simulink model "Strategia_pilotaggio_XY"  (R2020b)
settings: Solver=VariableStepAuto  StartTime=0.0  StopTime=tsim  RelTol=1e-3
values from neighbouring files (symbols this model uses):
  Acc_asse_x = []    [main_Strategia_di_pilotaggio.m]
  Acc_asse_y = []    [main_Strategia_di_pilotaggio.m]
  mx = config_dc_x(parx)    [Main_traiettoria.m]    (also in Main_traiettoria_ordinato.m; main_Strategia_di_pilotaggio.m)
  my = config_dc_y(pary)    [Main_traiettoria.m]    (also in Main_traiettoria_ordinato.m; main_Strategia_di_pilotaggio.m)
  time = 0:tf/np:tf    [Main_traiettoria.m]    (also in Main_traiettoria_ordinato.m = 0:passo:tsim)
  Vel_asse_x = []    [main_Strategia_di_pilotaggio.m]
  Vel_asse_y = []    [main_Strategia_di_pilotaggio.m]
  x = zeros(length(time),1)    [Main_traiettoria.m]    (also in Main_traiettoria_ordinato.m; main_Strategia_di_pilotaggio.m = [])
  y = zeros(length(time),1)    [Main_traiettoria.m]    (also in Main_traiettoria_ordinato.m; main_Strategia_di_pilotaggio.m = [])
undefined symbols (not defined in the file or in its folder): accelerazioni, accelerazioniy, ci_x, ci_y, Evaluate_Trajectory, interpolazione_tempi, parx, pary
libraries: cstblocks x16, simulink x3
settings Model: Creator=stefa  LastModifiedBy=user
settings DebuggingCC: SFMachineParentedDataDiag=error

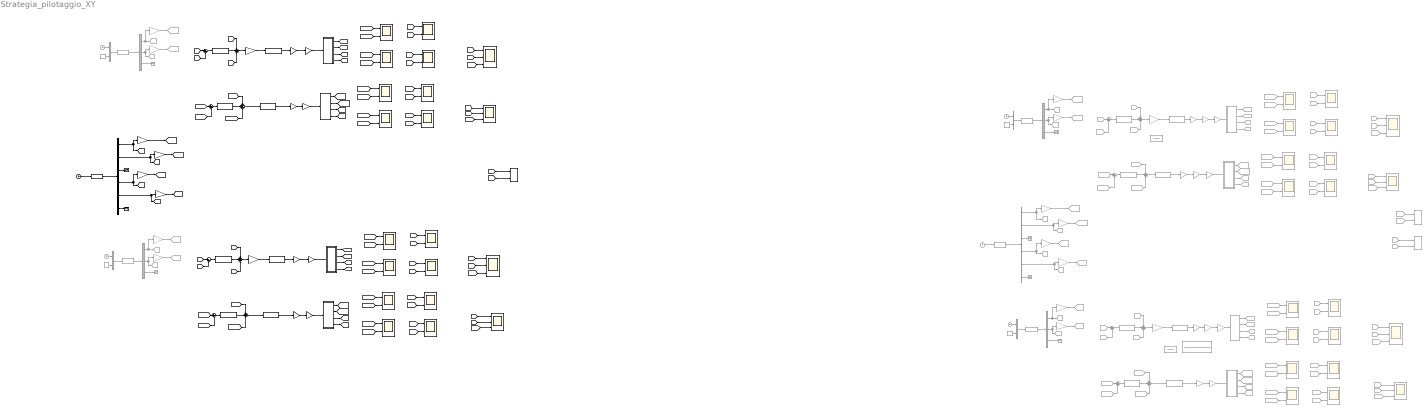
== system Strategia_pilotaggio_XY ==
  note: Vel carrello confronto
  note: Retroazione Motore
  note: Retroazione Motore
  note: Grafici
  note: Grafici
  note: Retroazione carrello
  note: ASSE "X"
  note: Pos carrello confronto
  note: Retroazione carrello
  note: Pos carrello confronto
  note: ASSE "Y"
  note: Vel carrello confronto
  note: ASSE "XY"
  note: Retroazione Motore
  note: Grafici
  note: Vel carrello confronto
  note: Grafici
  note: ASSE "Y"
  note: Pos carrello confronto
  note: Retroazione Motore
  note: Retroazione carrello
  note: Pos carrello confronto
  note: Retroazione carrello
  note: ASSE "XY"
  note: Vel carrello confronto
  note: ASSE "X"
   {1..2,5..8} (6 alike) : Terminator  Commented=on
  " 3" : Terminator
  " 4" : Terminator
  Constant{1..4} (4 alike) : Constant  Commented=on  Value=0.6
  Demux{1..2,4..5} (4 alike) : Demux  Commented=on  Outputs=3
  Demux3 : Demux  Outputs=6
  Demux6 : Demux  Commented=on  Outputs=6
  Discrete Filter1 : DiscreteFilter  Commented=on  Denominator=[1 0.7]
  Discrete Filter2 : DiscreteFilter  Commented=on  Denominator=[1 0.3]
  Discrete Filter3 : DiscreteFilter  Commented=on  Denominator=[(2*pi*150)^2 (2*pi*150/0.8) 1]
  From{100,107,110,119} (4 alike) : From  Commented=on  GotoTag=y
  From101 : From  Commented=on  GotoTag=theta1_ref
  From102 : From  Commented=on  GotoTag=theta1_rifmot
  From103 : From  Commented=on  GotoTag=theta1p_ref
  From104 : From  Commented=on  GotoTag=theta1p_rifmot
  From{87,98,105,112} (4 alike) : From  Commented=on  GotoTag=y_ref
  From{63,73,81,106} (4 alike) : From  Commented=on  GotoTag=x_ref
  From{99,108,114..115} (4 alike) : From  Commented=on  GotoTag=yp_ref
  From109 : From  Commented=on  GotoTag=yp
  From111 : From  Commented=on  GotoTag=yp_rifmot
  From113 : From  Commented=on  GotoTag=y_rifmot
  From116 : From  Commented=on  GotoTag=x_rifmot
  From117 : From  Commented=on  GotoTag=yp
  From{76,82,96,118} (4 alike) : From  Commented=on  GotoTag=x
  From{75,83,120..121} (4 alike) : From  Commented=on  GotoTag=xp_ref
  From122 : From  Commented=on  GotoTag=xp
  From123 : From  Commented=on  GotoTag=xp
  From124 : From  Commented=on  GotoTag=theta1p_rifmotx
  From125 : From  Commented=on  GotoTag=yp
  From126 : From  Commented=on  GotoTag=theta1p_rifmot
  From64 : From  Commented=on  GotoTag=xp_rifmot
  From65 : From  Commented=on  GotoTag=theta1_refx
  From66 : From  Commented=on  GotoTag=theta1p_refx
  From67 : From  Commented=on  GotoTag=theta1_rifmotx
  From68 : From  Commented=on  GotoTag=theta1_refx
  From69 : From  Commented=on  GotoTag=theta1x
  From70 : From  Commented=on  GotoTag=theta1p_refx
  From71 : From  Commented=on  GotoTag=theta1px
  From72 : From  Commented=on  GotoTag=x_rifmot
  From74 : From  Commented=on  GotoTag=x_rifmot
  From77 : From  Commented=on  GotoTag=theta1_refx
  From78 : From  Commented=on  GotoTag=theta1_rifmotx
  From79 : From  Commented=on  GotoTag=theta1p_refx
  From80 : From  Commented=on  GotoTag=theta1p_rifmotx
  From84 : From  Commented=on  GotoTag=xp
  From85 : From  Commented=on  GotoTag=y_rifmot
  From86 : From  Commented=on  GotoTag=xp_rifmot
  From88 : From  Commented=on  GotoTag=yp_rifmot
  From89 : From  Commented=on  GotoTag=theta1_ref
  From90 : From  Commented=on  GotoTag=theta1p_ref
  From91 : From  Commented=on  GotoTag=theta1_rifmot
  From92 : From  Commented=on  GotoTag=theta1_ref
  From93 : From  Commented=on  GotoTag=theta1
  From94 : From  Commented=on  GotoTag=theta1p_ref
  From95 : From  Commented=on  GotoTag=theta1p
  From97 : From  Commented=on  GotoTag=y_rifmot
  G-agg : Gain  Commented=on  Gain=0.09
  G_AGG : Gain  Commented=on  Gain=0.5
  G_AGG1 : Gain  Commented=on  Gain=0.19
  Gain{1,4,11,13,15,18..19} (7 alike) : Gain  Commented=on  Gain=1/parx.tau
  Gain10 : Gain  Gain=1/pary.tau
  Gain{3,6,12,14,16..17,20} (7 alike) : Gain  Commented=on  Gain=1/pary.tau
  Gain2 : Gain  Gain=1/parx.tau
  Gain5 : Gain  Gain=1/pary.tau
  Gain7 : Gain  Gain=1/parx.tau
  Gain8 : Gain  Gain=1/parx.tau
  Gain9 : Gain  Gain=1/pary.tau
  Goto11 : Goto  Commented=on  GotoTag=xp_ref
  Goto14 : Goto  Commented=on  GotoTag=yp_ref
  Goto18 : Goto  Commented=on  GotoTag=theta1_ref
  Goto2 : Goto  Commented=on  GotoTag=theta1_refx
  Goto20 : Goto  Commented=on  GotoTag=theta1p_ref
  Goto23 : Goto  Commented=on  GotoTag=y_ref
  Goto33 : Goto  Commented=on  GotoTag=xp_rifmot
  Goto34 : Goto  Commented=on  GotoTag=xp
  Goto35 : Goto  Commented=on  GotoTag=xp_ref
  Goto36 : Goto  Commented=on  GotoTag=yp
  Goto37 : Goto  Commented=on  GotoTag=theta1p_rifmotx
  Goto38 : Goto  Commented=on  GotoTag=yp_ref
  Goto39 : Goto  Commented=on  GotoTag=x
  Goto4 : Goto  Commented=on  GotoTag=theta1p_refx
  Goto40 : Goto  Commented=on  GotoTag=theta1p_rifmot
  Goto41 : Goto  Commented=on  GotoTag=y
  Goto42 : Goto  Commented=on  GotoTag=theta1_ref
  Goto43 : Goto  Commented=on  GotoTag=y_rifmot
  Goto44 : Goto  Commented=on  GotoTag=theta1_refx
  Goto45 : Goto  Commented=on  GotoTag=theta1p_ref
  Goto46 : Goto  Commented=on  GotoTag=theta1p
  Goto47 : Goto  Commented=on  GotoTag=theta1
  Goto48 : Goto  Commented=on  GotoTag=y_ref
  Goto49 : Goto  Commented=on  GotoTag=theta1_rifmot
  Goto50 : Goto  Commented=on  GotoTag=xp_ref
  Goto51 : Goto  Commented=on  GotoTag=theta1_refx
  Goto52 : Goto  Commented=on  GotoTag=theta1p_refx
  Goto53 : Goto  Commented=on  GotoTag=x_ref
  Goto54 : Goto  Commented=on  GotoTag=yp_ref
  Goto55 : Goto  Commented=on  GotoTag=x_rifmot
  Goto56 : Goto  Commented=on  GotoTag=theta1_ref
  Goto57 : Goto  Commented=on  GotoTag=theta1p_ref
  Goto58 : Goto  Commented=on  GotoTag=y_ref
  Goto59 : Goto  Commented=on  GotoTag=theta1p_refx
  Goto60 : Goto  Commented=on  GotoTag=theta1px
  Goto61 : Goto  Commented=on  GotoTag=theta1x
  Goto62 : Goto  Commented=on  GotoTag=yp_rifmot
  Goto63 : Goto  Commented=on  GotoTag=x_ref
  Goto64 : Goto  Commented=on  GotoTag=theta1_rifmotx
  Goto8 : Goto  Commented=on  GotoTag=x_ref
  Km : Gain  Gain=mx.K
  Km1 : Gain  Gain=my.K
  Km2 : Gain  Commented=on  Gain=mx.K
  Km3 : Gain  Commented=on  Gain=my.K
  Kr : Gain  Gain=mx.Kr
  Kr1 : Gain  Gain=mx.Kr
  Kr2 : Gain  Gain=my.Kr
  Kr3 : Gain  Gain=my.Kr
  Kr4 : Gain  Commented=on  Gain=mx.Kr
  Kr5 : Gain  Commented=on  Gain=mx.Kr
  Kr6 : Gain  Commented=on  Gain=my.Kr
  Kr7 : Gain  Commented=on  Gain=my.Kr
  Mux{1..4} (4 alike) : Mux  Commented=on  Inputs=2
  Pos. Motore con retr. Mot : Scope  NumInputPorts=2
  Pos. Motore con retr. Mot1 : Scope  NumInputPorts=2
  Pos. Motore con retr. Mot2 : Scope  Commented=on  NumInputPorts=2
  Pos. Motore con retr. Mot3 : Scope  Commented=on  NumInputPorts=2
  Pos. Motore con retr. carrello : Scope  NumInputPorts=2
  Pos. Motore con retr. carrello1 : Scope  NumInputPorts=2
  Pos. Motore con retr. carrello2 : Scope  Commented=on  NumInputPorts=2
  Pos. Motore con retr. carrello3 : Scope  Commented=on  NumInputPorts=2
  Pos. carrello con retr. Mot : Scope  NumInputPorts=2
  Pos. carrello con retr. Mot1 : Scope  NumInputPorts=2
  Pos. carrello con retr. Mot2 : Scope  Commented=on  NumInputPorts=2
  Pos. carrello con retr. Mot3 : Scope  Commented=on  NumInputPorts=2
  Pos. carrello con retr. carrello : Scope  NumInputPorts=2
  Pos. carrello con retr. carrello1 : Scope  NumInputPorts=2
  Pos. carrello con retr. carrello2 : Scope  Commented=on  NumInputPorts=2
  Pos. carrello con retr. carrello3 : Scope  Commented=on  NumInputPorts=2
  Pos. carrello confronto : Scope  NumInputPorts=3
  Pos. carrello confronto1 : Scope  NumInputPorts=3
  Pos. carrello confronto2 : Scope  Commented=on  NumInputPorts=3
  Pos. carrello confronto3 : Scope  Commented=on  NumInputPorts=3
  REGOLATORE POSIZIONE1 : cstblocks/LTI System  sys=apx.H_P  IC=[]
  REGOLATORE POSIZIONE2 : cstblocks/LTI System  sys=apx.H_P  IC=[]
  REGOLATORE POSIZIONE3 : cstblocks/LTI System  sys=apy.H_P  IC=[]
  REGOLATORE POSIZIONE4 : cstblocks/LTI System  sys=apy.H_P  IC=[]
  REGOLATORE POSIZIONE5 : cstblocks/LTI System  Commented=on  sys=apx.H_P  IC=[]
  REGOLATORE POSIZIONE6 : cstblocks/LTI System  Commented=on  sys=apx.H_P  IC=[]
  REGOLATORE POSIZIONE7 : cstblocks/LTI System  Commented=on  sys=apy.H_P  IC=[]
  REGOLATORE POSIZIONE8 : cstblocks/LTI System  Commented=on  sys=apy.H_P  IC=[]
  REGOLATORE VELOCITA1 : cstblocks/LTI System  sys=avx.PI_V  IC=[]
  REGOLATORE VELOCITA2 : cstblocks/LTI System  sys=avx.PI_V  IC=[]
  REGOLATORE VELOCITA3 : cstblocks/LTI System  sys=avy.PI_V  IC=[]
  REGOLATORE VELOCITA4 : cstblocks/LTI System  sys=avy.PI_V  IC=[]
  REGOLATORE VELOCITA5 : cstblocks/LTI System  Commented=on  sys=avx.PI_V  IC=[]
  REGOLATORE VELOCITA6 : cstblocks/LTI System  Commented=on  sys=avx.PI_V  IC=[]
  REGOLATORE VELOCITA7 : cstblocks/LTI System  Commented=on  sys=avy.PI_V  IC=[]
  REGOLATORE VELOCITA8 : cstblocks/LTI System  Commented=on  sys=avy.PI_V  IC=[]
  Sum{1..2,5..6} (4 alike) : Sum  Inputs=|+-
  Sum{9..10,13..14} (4 alike) : Sum  Commented=on  Inputs=|+-
  Sum{11..12,15..16} (4 alike) : Sum  Commented=on  Inputs=++-
  Sum{3..4,7..8} (4 alike) : Sum  Inputs=++-
  Vel. Motore con retr. Mot : Scope  NumInputPorts=2
  Vel. Motore con retr. Mot1 : Scope  NumInputPorts=2
  Vel. Motore con retr. Mot2 : Scope  Commented=on  NumInputPorts=2
  Vel. Motore con retr. Mot3 : Scope  Commented=on  NumInputPorts=2
  Vel. Motore con retr. carrello : Scope  NumInputPorts=2
  Vel. Motore con retr. carrello1 : Scope  NumInputPorts=2
  Vel. Motore con retr. carrello2 : Scope  Commented=on  NumInputPorts=2
  Vel. Motore con retr. carrello3 : Scope  Commented=on  NumInputPorts=2
  Vel. carrello con retr. Mot : Scope  NumInputPorts=2
  Vel. carrello con retr. Mot1 : Scope  NumInputPorts=2
  Vel. carrello con retr. Mot2 : Scope  Commented=on  NumInputPorts=2
  Vel. carrello con retr. Mot3 : Scope  Commented=on  NumInputPorts=2
  Vel. carrello con retr. carrello : Scope  NumInputPorts=2
  Vel. carrello con retr. carrello1 : Scope  NumInputPorts=2
  Vel. carrello con retr. carrello2 : Scope  Commented=on  NumInputPorts=2
  Vel. carrello con retr. carrello3 : Scope  Commented=on  NumInputPorts=2
  Vel. carrello confronto : Scope  NumInputPorts=3
  Vel. carrello confronto1 : Scope  NumInputPorts=3
  Vel. carrello confronto2 : Scope  Commented=on  NumInputPorts=3
  Vel. carrello confronto3 : Scope  Commented=on  NumInputPorts=3
  XY Graph : simulink/Sinks/XY Graph  xmin=-1  xmax=1  ymin=-1  ymax=1  st=-1
  XY Graph1 : simulink/Sinks/XY Graph  Commented=on  xmin=-0.5  xmax=0.3  ymin=-0.5  ymax=0.3  st=-1
  XY Graph2 : simulink/Sinks/XY Graph  Commented=on  xmin=-0.5  xmax=0.3  ymin=-0.5  ymax=0.3  st=-1
  blocco 4 gdl1 : Subsystem
  blocco 4 gdl2 : Subsystem
  blocco 4 gdl3 : Subsystem
  blocco 4 gdl4 : Subsystem
  blocco 4 gdl5 : Subsystem  Commented=on
  blocco 4 gdl6 : Subsystem  Commented=on
  blocco 4 gdl7 : Subsystem  Commented=on
  blocco 4 gdl8 : Subsystem  Commented=on
  chopper1 : Gain  Gain=my.K
  chopper2 : Gain  Gain=mx.K
  chopper3 : Gain  Commented=on  Gain=my.K
  chopper4 : Gain  Commented=on  Gain=mx.K
  generatore profilo moto{1..2,4..5} (4 alike) : MATLABFcn  Commented=on  MATLABFcn=Evaluate_Trajectory( u(1) , u(2))  OutputDimensions=3
  generatore profilo moto3 : MATLABFcn  MATLABFcn=interpolazione_tempi(x,Vel_asse_x,Acc_asse_x,y,Vel_asse_y,Acc_asse_y,u,time)  OutputDimensions=6
  generatore profilo moto6 : MATLABFcn  Commented=on  MATLABFcn=interpolazione_tempi(x,Vel_asse_x,Acc_asse_x,y,Vel_asse_y,Acc_asse_y,u,time)  OutputDimensions=6
  tempo{1..2,4..6} (5 alike) : Clock  Commented=on
      tempo6 settings: Decimation=tsim
  tempo3 : Clock
      settings: Decimation=tsim
  wires:
  [y] -> XY Graph/2  "y retr. carrello"
  [theta1p] -> Vel. Motore con retr. carrello1/2  "theta1p"
  Mux2/1 -> generatore profilo moto1/1
  [theta1p_ref] -> Vel. Motore con retr. carrello1/1  "thehta1p_ref"
  Mux1/1 -> generatore profilo moto2/1
  [theta1_rifmot] -> Sum5/2
  blocco 4 gdl4/2(Out1) -> [theta1p_rifmot]
  [xp] -> Vel. carrello confronto/2  "xp_retcarr"
  Demux3/2 -> Gain7/1, [xp_ref]  "XP"
  [yp_rifmot] -> Vel. carrello con retr. Mot1/2  "yp"
  [theta1p_refx] -> Vel. Motore con retr. Mot/1  "theta1p_ref"
  tempo1/1 -> Mux2/1
  blocco 4 gdl3/1(Out2) -> [theta1]
  Demux3/5 -> Gain9/1, [yp_ref]  "YP"
  [yp_ref] -> Sum7/1
  [x] -> XY Graph/1  "x_retcarr"
  Gain10/1 -> [theta1_ref]  "motore"
  [theta1p_rifmot] -> Vel. Motore con retr. Mot1/2  "theta1p"
  [theta1p_ref] -> Sum8/1
  [y_ref] -> Pos. carrello con retr. carrello1/1  "y_ref"
  Demux3/3 -> " 3"/1  "XPP"
  Demux1/2 -> Gain3/1, Goto14/1  "YP"
  Gain9/1 -> [theta1p_ref]  "motore"
  tempo3/1 -> generatore profilo moto3/1
  Demux3/4 -> Gain10/1, [y_ref]  "Y"
  Demux3/6 -> " 4"/1  "YPP"
  Km1/1 -> blocco 4 gdl3/1(In1)  "Cm"
  [x_ref] -> Pos. carrello con retr. carrello/1  "x_ref"
  [y_rifmot] -> Pos. carrello con retr. Mot1/2  "y"
  blocco 4 gdl4/3(Out3) -> [y_rifmot]
  blocco 4 gdl2/2(Out4) -> [theta1p_rifmotx]
  blocco 4 gdl3/2(Out1) -> [theta1p]
  [theta1_rifmot] -> Pos. Motore con retr. Mot1/2  "theta1"
  [y_ref] -> Pos. carrello con retr. Mot1/1  "y_ref"
  Kr2/1 -> Km1/1  "I"
  [y_ref] -> Pos. carrello confronto1/1  "y ldm"
  Gain8/1 -> [theta1_refx]  "motore"
  Demux3/1 -> Gain8/1, [x_ref]  "X"
  Gain7/1 -> [theta1p_refx]  "motore"
  REGOLATORE POSIZIONE4/1 -> Sum8/2
  [y] -> Sum6/2
  [theta1_rifmotx] -> Pos. Motore con retr. Mot/2  "theta1"
  [theta1_ref] -> Pos. Motore con retr. carrello1/1  "theta1_ref"
  [theta1_rifmotx] -> Sum1/2
  blocco 4 gdl3/3(Out3) -> [y]
  [y] -> Pos. carrello con retr. carrello1/2  "y"
  Constant1/1 -> Mux1/2
  Sum3/1 -> Gain2/1
  [yp] -> Sum7/3
  [y_ref] -> Sum6/1
  blocco 4 gdl4/1(Out2) -> [theta1_rifmot]
  Sum5/1 -> REGOLATORE POSIZIONE4/1
  [x] -> Pos. carrello confronto/2  "x_retcarr"
  Gain3/1 -> Goto20/1  "motore"
  blocco 4 gdl1/4(Out8) -> [xp]
  [theta1p_rifmot] -> Sum8/3
  [yp_ref] -> Vel. carrello con retr. Mot1/1  "yp_ref"
  Constant2/1 -> Mux2/2
  REGOLATORE POSIZIONE3/1 -> Sum7/2
  Gain6/1 -> Goto18/1  "motore"
  [yp_ref] -> Vel. carrello con retr. carrello1/1  "yp_ref"
  [xp_ref] -> Vel. carrello con retr. carrello/1  "xp_ref"
  Sum6/1 -> REGOLATORE POSIZIONE3/1
  [theta1_refx] -> Sum1/1
  [yp] -> Vel. carrello con retr. carrello1/2  "yp"
  [xp_ref] -> Vel. carrello con retr. Mot/1  "xp_ref"
  REGOLATORE VELOCITA4/1 -> Kr2/1  "Va"
  REGOLATORE VELOCITA3/1 -> Kr3/1  "Va"
  Sum8/1 -> REGOLATORE VELOCITA3/1
  [yp_rifmot] -> Vel. carrello confronto1/3  "yp retr. motore"
  generatore profilo moto1/1 -> Demux1/1  "carrello"
  [xp_rifmot] -> Vel. carrello confronto/3  "xp_retmot"
  blocco 4 gdl3/4(Out4) -> [yp]
  [theta1x] -> Pos. Motore con retr. carrello/2  "tetha1"
  [y] -> Pos. carrello confronto1/2  "y retr. carrello"
  [xp] -> Sum3/3
  [theta1p_ref] -> Vel. Motore con retr. Mot1/1  "thehta1p_ref"
  Demux1/3 -> " 2"/1  "YPP"
  blocco 4 gdl1/1(Out3) -> [theta1x]
  Gain5/1 -> REGOLATORE VELOCITA4/1  "theta1_rif"
  chopper2/1 -> blocco 4 gdl2/1(In1)  "Cm"
  [theta1] -> Pos. Motore con retr. carrello1/2  "theta1"
  blocco 4 gdl1/3(Out7) -> [x]
  Gain1/1 -> Goto4/1  "motore"
  [x_ref] -> Pos. carrello confronto/1  "x_ref"
  [xp_ref] -> Vel. carrello confronto/1  "xp_ref"
  Gain4/1 -> Goto2/1  "motore"
  Sum1/1 -> REGOLATORE POSIZIONE2/1
  [theta1p_rifmotx] -> Sum4/3
  [x_ref] -> Pos. carrello con retr. Mot/1  "x"
  REGOLATORE POSIZIONE2/1 -> Sum4/2
  [x_rifmot] -> Pos. carrello con retr. Mot/2  "x_rif"
  [theta1_refx] -> Pos. Motore con retr. carrello/1  "theta1_ref"
  REGOLATORE VELOCITA1/1 -> Kr1/1  "Va"
  [theta1p_rifmotx] -> Vel. Motore con retr. Mot/2  "theta1p"
  [theta1p_refx] -> Vel. Motore con retr. carrello/1  "theta1p_ref"
  Km/1 -> blocco 4 gdl1/1(In1)  "Cm"
  [x] -> Sum2/2
  [theta1_refx] -> Pos. Motore con retr. Mot/1  "theta1_ref"
  Demux2/2 -> Gain1/1, Goto11/1  "XP"
  Sum7/1 -> Gain5/1
  blocco 4 gdl1/2(Out4) -> [theta1px]
  [xp] -> Vel. carrello con retr. carrello/2  "xp"
  [x_ref] -> Sum2/1
  Demux2/1 -> Goto8/1, Gain4/1  "X"
  [theta1_ref] -> Pos. Motore con retr. Mot1/1  "theta1_ref"
  generatore profilo moto2/1 -> Demux2/1  "carrello"
  [theta1px] -> Vel. Motore con retr. carrello/2  "thehta1p"
  tempo2/1 -> Mux1/1
  Gain2/1 -> REGOLATORE VELOCITA2/1  "theta1_rifx"
  generatore profilo moto3/1 -> Demux3/1  "carrello"
  [yp] -> Vel. carrello confronto1/2  "yp retr. carrello"
  Kr1/1 -> chopper2/1  "I"
  Demux2/3 -> " 1"/1  "XPP"
  [xp_ref] -> Sum3/1
  Kr/1 -> Km/1  "I"
  Sum4/1 -> REGOLATORE VELOCITA1/1
  REGOLATORE POSIZIONE1/1 -> Sum3/2
  REGOLATORE VELOCITA2/1 -> Kr/1  "Va"
  [theta1p_refx] -> Sum4/1
  blocco 4 gdl2/3(Out7) -> [x_rifmot]
  blocco 4 gdl2/4(Out1) -> [xp_rifmot]
  Kr3/1 -> chopper1/1  "I"
  [yp_ref] -> Vel. carrello confronto1/1  "yp ldm"
  blocco 4 gdl2/1(Out3) -> [theta1_rifmotx]
  Demux1/1 -> Goto23/1, Gain6/1  "Y"
  blocco 4 gdl4/4(Out4) -> [yp_rifmot]
  [x_rifmot] -> Pos. carrello confronto/3  "x_retmot"
  chopper1/1 -> blocco 4 gdl4/1(In1)  "Cm"
  [y_rifmot] -> Pos. carrello confronto1/3  "y retr. motore"
  [x] -> Pos. carrello con retr. carrello/2  "x"
  [xp_rifmot] -> Vel. carrello con retr. Mot/2  "xp"
  Sum2/1 -> REGOLATORE POSIZIONE1/1
  [theta1_ref] -> Sum5/1
  From109/1 -> Vel. carrello confronto3/2  "yp retr. carrello"
  From106/1 -> Pos. carrello con retr. Mot2/1  "x"
  From77/1 -> Pos. Motore con retr. Mot2/1  "theta1_ref"
  Gain13/1 -> REGOLATORE VELOCITA6/1  "theta1_rifx"
  Kr5/1 -> chopper4/1  "I"
  REGOLATORE POSIZIONE8/1 -> Sum16/2
  REGOLATORE VELOCITA8/1 -> G-agg/1  "Va"
  Demux5/2 -> Gain11/1, Goto35/1  "XP"
  blocco 4 gdl5/2(Out4) -> Goto60/1
  From70/1 -> Vel. Motore con retr. carrello2/1  "theta1p_ref"
  From101/1 -> Pos. Motore con retr. Mot3/1  "theta1_ref"
  Demux5/1 -> Goto63/1, Gain15/1  "X"
  From63/1 -> Sum10/1
  blocco 4 gdl7/4(Out4) -> Goto36/1
  From89/1 -> Sum13/1
  Sum16/1 -> REGOLATORE VELOCITA7/1
  From64/1 -> Vel. carrello con retr. Mot2/2  "xp"
  chopper3/1 -> blocco 4 gdl8/1(In1)  "Cm"
  blocco 4 gdl6/3(Out7) -> Goto55/1
  From82/1 -> Pos. carrello con retr. carrello2/2  "x"
  From97/1 -> Pos. carrello confronto3/3  "y retr. motore"
  From105/1 -> Pos. carrello con retr. carrello3/1  "y_ref"
  From113/1 -> Pos. carrello con retr. Mot3/2  "y"
  From81/1 -> Pos. carrello con retr. carrello2/1  "x_ref"
  tempo6/1 -> generatore profilo moto6/1
  Demux4/2 -> Gain14/1, Goto38/1  "YP"
  From90/1 -> Sum16/1
  From87/1 -> Sum14/1
  Kr6/1 -> Km3/1  "I"
  Sum11/1 -> Gain13/1
  Constant3/1 -> Mux3/2
  From98/1 -> Pos. carrello confronto3/1  "y ldm"
  Gain18/1 -> Goto52/1  "motore"
  From92/1 -> Pos. Motore con retr. carrello3/1  "theta1_ref"
  Gain19/1 -> Goto51/1  "motore"
  From102/1 -> Pos. Motore con retr. Mot3/2  "theta1"
  Demux6/1 -> Gain19/1, Goto53/1  "X"
  blocco 4 gdl6/2(Out4) -> Goto37/1
  Kr4/1 -> Km2/1  "I"
  From75/1 -> Sum11/1
  From117/1 -> Vel. carrello con retr. carrello3/2  "yp"
  Gain11/1 -> Goto59/1  "motore"
  blocco 4 gdl6/1(Out3) -> Goto64/1
  Sum15/1 -> Gain16/1
  G_AGG1/1 -> Kr4/1  "I"
  generatore profilo moto5/1 -> Demux5/1  "carrello"
  From85/1 -> XY Graph2/2  "y retr. motore"
  blocco 4 gdl7/3(Out3) -> Goto41/1
  generatore profilo moto6/1 -> Demux6/1  "carrello"
  From112/1 -> Pos. carrello con retr. Mot3/1  "y_ref"
  From121/1 -> Vel. carrello con retr. carrello2/1  "xp_ref"
  REGOLATORE VELOCITA5/1 -> G_AGG/1  "Va"
  From83/1 -> Vel. carrello confronto2/1  "xp_ref"
  From74/1 -> XY Graph2/1  "x_retmot"
  blocco 4 gdl8/3(Out3) -> Goto43/1
  REGOLATORE VELOCITA6/1 -> G_AGG1/1  "Va"
  Gain16/1 -> REGOLATORE VELOCITA8/1  "theta1_rif"
  chopper4/1 -> blocco 4 gdl6/1(In1)  "Cm"
  Km3/1 -> blocco 4 gdl7/1(In1)  "Cm"
  From111/1 -> Vel. carrello confronto3/3  "yp retr. motore"
  G_AGG/1 -> Kr5/1  "I"
  Gain14/1 -> Goto45/1  "motore"
  From65/1 -> Sum9/1
  tempo5/1 -> Mux3/1
  From80/1 -> Vel. Motore con retr. Mot2/2  "theta1p"
  REGOLATORE POSIZIONE5/1 -> Sum11/2
  Gain20/1 -> Goto57/1  "motore"
  From115/1 -> Vel. carrello con retr. carrello3/1  "yp_ref"
  blocco 4 gdl8/4(Out4) -> Goto62/1
  From71/1 -> Vel. Motore con retr. carrello2/2  "thehta1p"
  Demux6/6 -> " 8"/1  "YPP"
  From103/1 -> Vel. Motore con retr. Mot3/1  "thehta1p_ref"
  REGOLATORE VELOCITA7/1 -> Kr7/1  "Va"
  REGOLATORE POSIZIONE7/1 -> Sum15/2
  Constant4/1 -> Mux4/2
  blocco 4 gdl8/1(Out2) -> Goto49/1
  Sum13/1 -> REGOLATORE POSIZIONE8/1
  From120/1 -> Vel. carrello con retr. Mot2/1  "xp_ref"
  From86/1 -> Vel. carrello confronto2/3  "xp_retmot"
  From78/1 -> Pos. Motore con retr. Mot2/2  "theta1"
  Km2/1 -> blocco 4 gdl5/1(In1)  "Cm"
  Sum14/1 -> REGOLATORE POSIZIONE7/1
  blocco 4 gdl6/4(Out1) -> Goto33/1
  Demux4/3 -> " 6"/1  "YPP"
  From93/1 -> Pos. Motore con retr. carrello3/2  "theta1"
  blocco 4 gdl5/3(Out7) -> Goto39/1
  Gain15/1 -> Goto44/1  "motore"
  blocco 4 gdl5/4(Out8) -> Goto34/1
  From73/1 -> Pos. carrello confronto2/1  "x_ref"
  Demux6/4 -> Gain12/1, Goto58/1  "Y"
  From68/1 -> Pos. Motore con retr. carrello2/1  "theta1_ref"
  From116/1 -> Pos. carrello con retr. Mot2/2  "x_rif"
  From69/1 -> Pos. Motore con retr. carrello2/2  "tetha1"
  From100/1 -> Pos. carrello confronto3/2  "y retr. carrello"
  Sum9/1 -> REGOLATORE POSIZIONE6/1
  G-agg/1 -> Kr6/1  "Cm"
  REGOLATORE POSIZIONE6/1 -> Sum12/2
  Sum10/1 -> REGOLATORE POSIZIONE5/1
  blocco 4 gdl7/2(Out1) -> Goto46/1
  Kr7/1 -> chopper3/1  "I"
  Demux6/3 -> " 7"/1  "XPP"
  From108/1 -> Vel. carrello confronto3/1  "yp ldm"
  blocco 4 gdl5/1(Out3) -> Goto61/1
  From84/1 -> Vel. carrello confronto2/2  "xp_retcarr"
  From107/1 -> Pos. carrello con retr. carrello3/2  "y"
  Sum12/1 -> REGOLATORE VELOCITA5/1
  From94/1 -> Vel. Motore con retr. carrello3/1  "thehta1p_ref"
  From114/1 -> Vel. carrello con retr. Mot3/1  "yp_ref"
  From76/1 -> Pos. carrello confronto2/2  "x_retcarr"
  Mux3/1 -> generatore profilo moto5/1
  From119/1 -> XY Graph1/2  "y retr. carrello"
  blocco 4 gdl8/2(Out1) -> Goto40/1
  Mux4/1 -> generatore profilo moto4/1
  From66/1 -> Sum12/1
  From72/1 -> Pos. carrello confronto2/3  "x_retmot"
  From104/1 -> Vel. Motore con retr. Mot3/2  "theta1p"
  Demux6/2 -> Gain18/1, Goto50/1  "XP"
  generatore profilo moto4/1 -> Demux4/1  "carrello"
  From95/1 -> Vel. Motore con retr. carrello3/2  "theta1p"
  Gain12/1 -> Goto56/1  "motore"
  Gain17/1 -> Goto42/1  "motore"
  From118/1 -> XY Graph1/1  "x_retcarr"
  blocco 4 gdl7/1(Out2) -> Goto47/1
  tempo4/1 -> Mux4/1
  Demux6/5 -> Gain20/1, Goto54/1  "YP"
  From122/1 -> Vel. carrello con retr. carrello2/2  "xp"
  From88/1 -> Vel. carrello con retr. Mot3/2  "yp"
  Demux5/3 -> " 5"/1  "XPP"
  From79/1 -> Vel. Motore con retr. Mot2/1  "theta1p_ref"
  Demux4/1 -> Goto48/1, Gain17/1  "Y"
  From99/1 -> Sum15/1
  From96/1 -> Sum10/2
  From123/1 -> Sum11/3
  From67/1 -> Sum9/2  "theta1_rifx"
  From124/1 -> Sum12/3  "theta1_rifx"
  From110/1 -> Sum14/2
  From125/1 -> Sum15/3
  From91/1 -> Sum13/2
  From126/1 -> Sum16/3

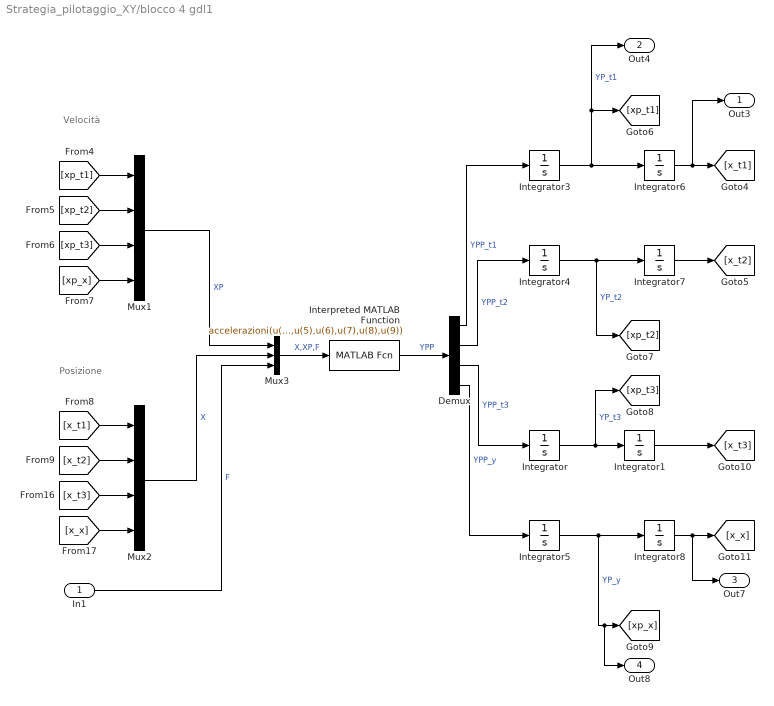
== system Strategia_pilotaggio_XY/blocco 4 gdl1 ==
  note: Velocità
  note: Posizione
  In1 : Inport
  Demux : Demux
  Integrator{,3..5} (4 alike) : Integrator
  Integrator1 : Integrator  InitialCondition=ci_x(3)
  Integrator6 : Integrator  InitialCondition=ci_x(1)
  Integrator7 : Integrator  InitialCondition=ci_x(2)
  Integrator8 : Integrator  InitialCondition=ci_x(4)
  Interpreted MATLAB Function : MATLABFcn  MATLABFcn=accelerazioni(u(1),u(2),u(3),u(4),u(5),u(6),u(7),u(8),u(9))  OutputDimensions=4
  Mux1 : Mux
  Mux2 : Mux
  Mux3 : Mux  Inputs=3
  Out3 : Outport
  Out4 : Outport  Port=2
  Out7 : Outport  Port=3
  Out8 : Outport  Port=4
  wires:
  Integrator4/1 -> [xp_t2], Integrator7/1  "YP_t2"
  [xp_t1] -> Mux1/1
  [x_t2] -> Mux2/2
  Integrator1/1 -> [x_t3]
  Demux/4 -> Integrator5/1  "YPP_y"
  Demux/2 -> Integrator4/1  "YPP_t2"
  In1/1 -> Mux3/3  "F"
  Mux3/1 -> Interpreted MATLAB Function/1  "X,XP,F"
  [xp_t2] -> Mux1/2
  Integrator6/1 -> Out3/1, [x_t1]
  Mux2/1 -> Mux3/2  "X"
  Demux/3 -> Integrator/1  "YPP_t3"
  Integrator5/1 -> Out8/1, [xp_x], Integrator8/1  "YP_y"
  Integrator8/1 -> Out7/1, [x_x]
  [xp_x] -> Mux1/4
  [x_x] -> Mux2/4
  Integrator7/1 -> [x_t2]
  Demux/1 -> Integrator3/1  "YPP_t1"
  [x_t1] -> Mux2/1
  Integrator3/1 -> Out4/1, [xp_t1], Integrator6/1  "YP_t1"
  [x_t3] -> Mux2/3
  Interpreted MATLAB Function/1 -> Demux/1  "YPP"
  Mux1/1 -> Mux3/1  "XP"
  Integrator/1 -> Integrator1/1, [xp_t3]  "YP_t3"
  [xp_t3] -> Mux1/3

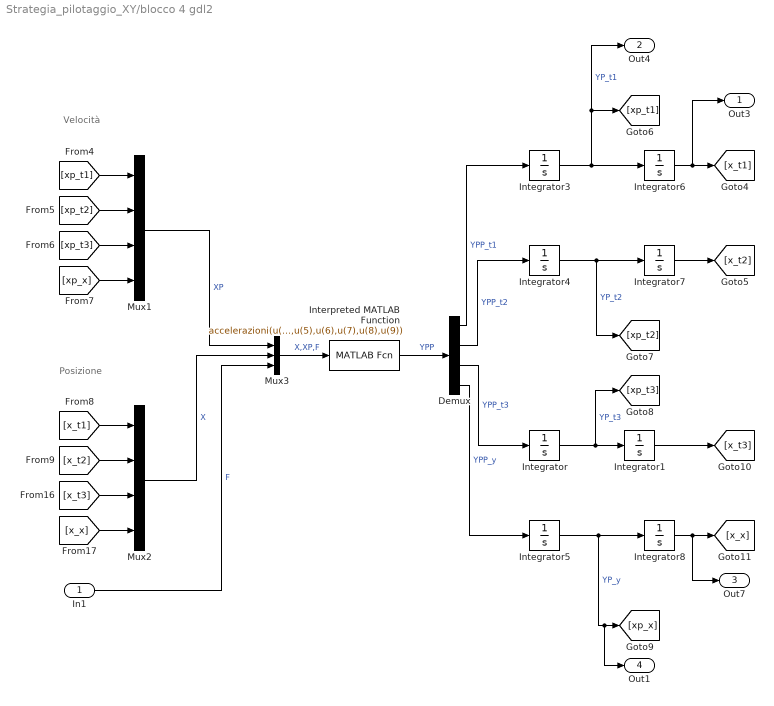
== system Strategia_pilotaggio_XY/blocco 4 gdl2 ==
  note: Posizione
  note: Velocità
  In1 : Inport
  Demux : Demux
  Integrator{,3..5} (4 alike) : Integrator
  Integrator1 : Integrator  InitialCondition=ci_x(3)
  Integrator6 : Integrator  InitialCondition=ci_x(1)
  Integrator7 : Integrator  InitialCondition=ci_x(2)
  Integrator8 : Integrator  InitialCondition=ci_x(4)
  Interpreted MATLAB Function : MATLABFcn  MATLABFcn=accelerazioni(u(1),u(2),u(3),u(4),u(5),u(6),u(7),u(8),u(9))  OutputDimensions=4
  Mux1 : Mux
  Mux2 : Mux
  Mux3 : Mux  Inputs=3
  Out3 : Outport
  Out4 : Outport  Port=2
  Out7 : Outport  Port=3
  Out1 : Outport  Port=4
  wires:
  [xp_t3] -> Mux1/3
  Interpreted MATLAB Function/1 -> Demux/1  "YPP"
  Integrator3/1 -> Out4/1, [xp_t1], Integrator6/1  "YP_t1"
  Integrator8/1 -> Out7/1, [x_x]
  Integrator7/1 -> [x_t2]
  [xp_x] -> Mux1/4
  [x_t1] -> Mux2/1
  Mux1/1 -> Mux3/1  "XP"
  [x_x] -> Mux2/4
  Demux/3 -> Integrator/1  "YPP_t3"
  Integrator/1 -> Integrator1/1, [xp_t3]  "YP_t3"
  Mux2/1 -> Mux3/2  "X"
  Integrator6/1 -> Out3/1, [x_t1]
  Integrator5/1 -> Out1/1, [xp_x], Integrator8/1  "YP_y"
  [xp_t2] -> Mux1/2
  Mux3/1 -> Interpreted MATLAB Function/1  "X,XP,F"
  [x_t3] -> Mux2/3
  In1/1 -> Mux3/3  "F"
  Demux/4 -> Integrator5/1  "YPP_y"
  Integrator4/1 -> [xp_t2], Integrator7/1  "YP_t2"
  Integrator1/1 -> [x_t3]
  [xp_t1] -> Mux1/1
  [x_t2] -> Mux2/2
  Demux/2 -> Integrator4/1  "YPP_t2"
  Demux/1 -> Integrator3/1  "YPP_t1"

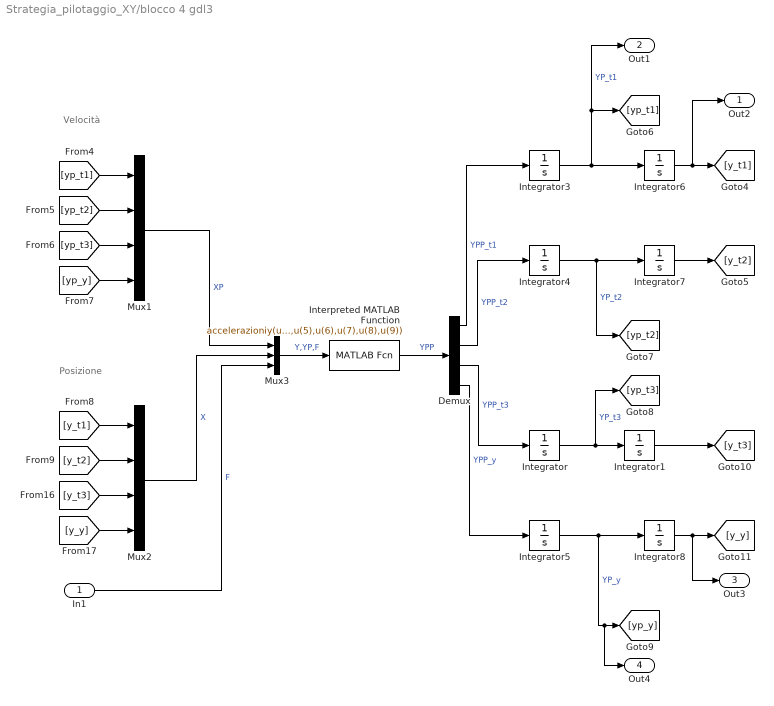
== system Strategia_pilotaggio_XY/blocco 4 gdl3 ==
  note: Posizione
  note: Velocità
  In1 : Inport
  Demux : Demux
  Integrator{,3..5} (4 alike) : Integrator
  Integrator1 : Integrator  InitialCondition=ci_y(3)
  Integrator6 : Integrator  InitialCondition=ci_y(1)
  Integrator7 : Integrator  InitialCondition=ci_y(2)
  Integrator8 : Integrator  InitialCondition=ci_y(4)
  Interpreted MATLAB Function : MATLABFcn  MATLABFcn=accelerazioniy(u(1),u(2),u(3),u(4),u(5),u(6),u(7),u(8),u(9))  OutputDimensions=4
  Mux1 : Mux
  Mux2 : Mux
  Mux3 : Mux  Inputs=3
  Out2 : Outport
  Out1 : Outport  Port=2
  Out3 : Outport  Port=3
  Out4 : Outport  Port=4
  wires:
  Integrator/1 -> Integrator1/1, [yp_t3]  "YP_t3"
  Mux1/1 -> Mux3/1  "XP"
  [y_t3] -> Mux2/3
  Mux3/1 -> Interpreted MATLAB Function/1  "Y,YP,F"
  [y_t2] -> Mux2/2
  Integrator7/1 -> [y_t2]
  Demux/3 -> Integrator/1  "YPP_t3"
  [yp_y] -> Mux1/4
  [y_y] -> Mux2/4
  Demux/1 -> Integrator3/1  "YPP_t1"
  [yp_t2] -> Mux1/2
  Mux2/1 -> Mux3/2  "X"
  Interpreted MATLAB Function/1 -> Demux/1  "YPP"
  Integrator8/1 -> Out3/1, [y_y]
  Integrator4/1 -> [yp_t2], Integrator7/1  "YP_t2"
  Integrator3/1 -> Out1/1, [yp_t1], Integrator6/1  "YP_t1"
  In1/1 -> Mux3/3  "F"
  Demux/2 -> Integrator4/1  "YPP_t2"
  Integrator5/1 -> Out4/1, [yp_y], Integrator8/1  "YP_y"
  Integrator6/1 -> Out2/1, [y_t1]
  [yp_t3] -> Mux1/3
  Demux/4 -> Integrator5/1  "YPP_y"
  Integrator1/1 -> [y_t3]
  [yp_t1] -> Mux1/1
  [y_t1] -> Mux2/1

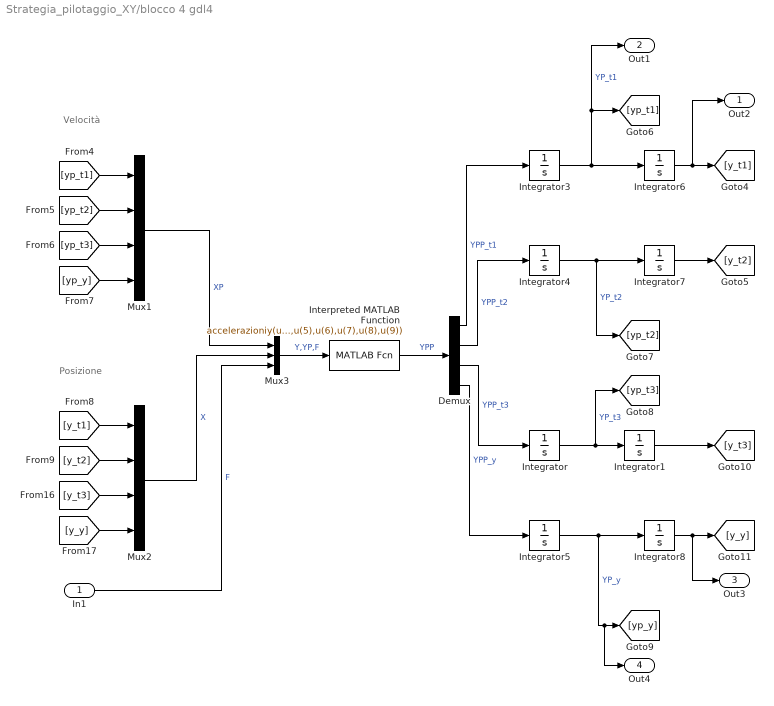
== system Strategia_pilotaggio_XY/blocco 4 gdl4 ==
  note: Posizione
  note: Velocità
  In1 : Inport
  Demux : Demux
  Integrator{,3..5} (4 alike) : Integrator
  Integrator1 : Integrator  InitialCondition=ci_y(3)
  Integrator6 : Integrator  InitialCondition=ci_y(1)
  Integrator7 : Integrator  InitialCondition=ci_y(2)
  Integrator8 : Integrator  InitialCondition=ci_y(4)
  Interpreted MATLAB Function : MATLABFcn  MATLABFcn=accelerazioniy(u(1),u(2),u(3),u(4),u(5),u(6),u(7),u(8),u(9))  OutputDimensions=4
  Mux1 : Mux
  Mux2 : Mux
  Mux3 : Mux  Inputs=3
  Out2 : Outport
  Out1 : Outport  Port=2
  Out3 : Outport  Port=3
  Out4 : Outport  Port=4
  wires:
  Integrator/1 -> Integrator1/1, [yp_t3]  "YP_t3"
  Mux1/1 -> Mux3/1  "XP"
  [y_t3] -> Mux2/3
  Mux3/1 -> Interpreted MATLAB Function/1  "Y,YP,F"
  [y_t2] -> Mux2/2
  Integrator7/1 -> [y_t2]
  Demux/3 -> Integrator/1  "YPP_t3"
  [yp_y] -> Mux1/4
  [y_y] -> Mux2/4
  Demux/1 -> Integrator3/1  "YPP_t1"
  [yp_t2] -> Mux1/2
  Mux2/1 -> Mux3/2  "X"
  Interpreted MATLAB Function/1 -> Demux/1  "YPP"
  Integrator8/1 -> Out3/1, [y_y]
  Integrator4/1 -> [yp_t2], Integrator7/1  "YP_t2"
  Integrator3/1 -> Out1/1, [yp_t1], Integrator6/1  "YP_t1"
  In1/1 -> Mux3/3  "F"
  Demux/2 -> Integrator4/1  "YPP_t2"
  Integrator5/1 -> Out4/1, [yp_y], Integrator8/1  "YP_y"
  Integrator6/1 -> Out2/1, [y_t1]
  [yp_t3] -> Mux1/3
  Demux/4 -> Integrator5/1  "YPP_y"
  Integrator1/1 -> [y_t3]
  [yp_t1] -> Mux1/1
  [y_t1] -> Mux2/1

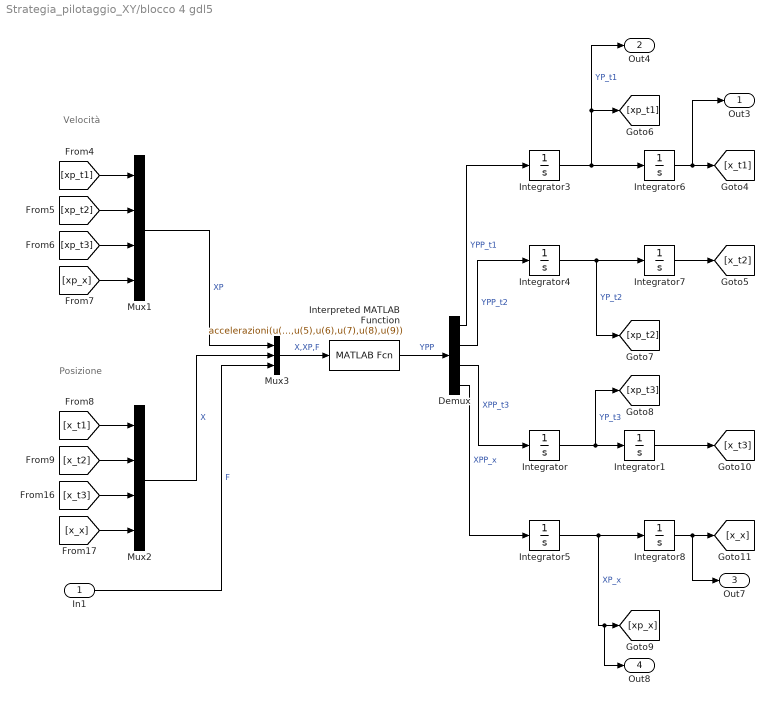
== system Strategia_pilotaggio_XY/blocco 4 gdl5 ==
  note: Velocità
  note: Posizione
  In1 : Inport
  Demux : Demux
  Integrator{,3..5} (4 alike) : Integrator
  Integrator1 : Integrator  InitialCondition=ci_x(3)
  Integrator6 : Integrator  InitialCondition=ci_x(1)
  Integrator7 : Integrator  InitialCondition=ci_x(2)
  Integrator8 : Integrator  InitialCondition=ci_x(4)
  Interpreted MATLAB Function : MATLABFcn  MATLABFcn=accelerazioni(u(1),u(2),u(3),u(4),u(5),u(6),u(7),u(8),u(9))  OutputDimensions=4
  Mux1 : Mux
  Mux2 : Mux
  Mux3 : Mux  Inputs=3
  Out3 : Outport
  Out4 : Outport  Port=2
  Out7 : Outport  Port=3
  Out8 : Outport  Port=4
  wires:
  Integrator4/1 -> [xp_t2], Integrator7/1  "YP_t2"
  [xp_t1] -> Mux1/1
  [x_t2] -> Mux2/2
  Integrator1/1 -> [x_t3]
  Demux/4 -> Integrator5/1  "XPP_x"
  Demux/2 -> Integrator4/1  "YPP_t2"
  In1/1 -> Mux3/3  "F"
  Mux3/1 -> Interpreted MATLAB Function/1  "X,XP,F"
  [xp_t2] -> Mux1/2
  Integrator6/1 -> Out3/1, [x_t1]
  Mux2/1 -> Mux3/2  "X"
  Demux/3 -> Integrator/1  "XPP_t3"
  Integrator5/1 -> Out8/1, [xp_x], Integrator8/1  "XP_x"
  Integrator8/1 -> Out7/1, [x_x]
  [xp_x] -> Mux1/4
  [x_x] -> Mux2/4
  Integrator7/1 -> [x_t2]
  Demux/1 -> Integrator3/1  "YPP_t1"
  [x_t1] -> Mux2/1
  Integrator3/1 -> Out4/1, [xp_t1], Integrator6/1  "YP_t1"
  [x_t3] -> Mux2/3
  Interpreted MATLAB Function/1 -> Demux/1  "YPP"
  Mux1/1 -> Mux3/1  "XP"
  Integrator/1 -> Integrator1/1, [xp_t3]  "YP_t3"
  [xp_t3] -> Mux1/3

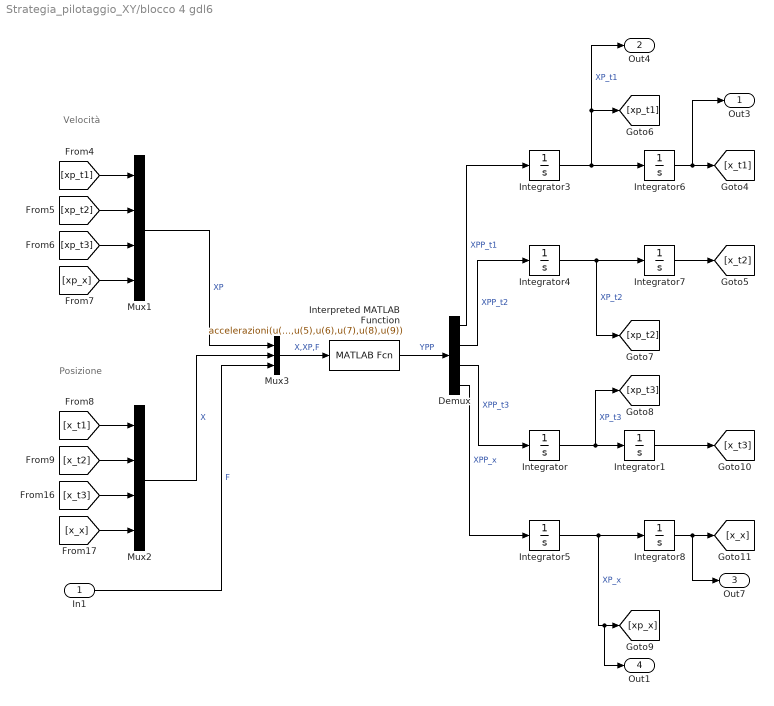
== system Strategia_pilotaggio_XY/blocco 4 gdl6 ==
  note: Posizione
  note: Velocità
  In1 : Inport
  Demux : Demux
  Integrator{,3..5} (4 alike) : Integrator
  Integrator1 : Integrator  InitialCondition=ci_x(3)
  Integrator6 : Integrator  InitialCondition=ci_x(1)
  Integrator7 : Integrator  InitialCondition=ci_x(2)
  Integrator8 : Integrator  InitialCondition=ci_x(4)
  Interpreted MATLAB Function : MATLABFcn  MATLABFcn=accelerazioni(u(1),u(2),u(3),u(4),u(5),u(6),u(7),u(8),u(9))  OutputDimensions=4
  Mux1 : Mux
  Mux2 : Mux
  Mux3 : Mux  Inputs=3
  Out3 : Outport
  Out4 : Outport  Port=2
  Out7 : Outport  Port=3
  Out1 : Outport  Port=4
  wires:
  [xp_t3] -> Mux1/3
  Interpreted MATLAB Function/1 -> Demux/1  "YPP"
  Integrator3/1 -> Out4/1, [xp_t1], Integrator6/1  "XP_t1"
  Integrator8/1 -> Out7/1, [x_x]
  Integrator7/1 -> [x_t2]
  [xp_x] -> Mux1/4
  [x_t1] -> Mux2/1
  Mux1/1 -> Mux3/1  "XP"
  [x_x] -> Mux2/4
  Demux/3 -> Integrator/1  "XPP_t3"
  Integrator/1 -> Integrator1/1, [xp_t3]  "XP_t3"
  Mux2/1 -> Mux3/2  "X"
  Integrator6/1 -> Out3/1, [x_t1]
  Integrator5/1 -> Out1/1, [xp_x], Integrator8/1  "XP_x"
  [xp_t2] -> Mux1/2
  Mux3/1 -> Interpreted MATLAB Function/1  "X,XP,F"
  [x_t3] -> Mux2/3
  In1/1 -> Mux3/3  "F"
  Demux/4 -> Integrator5/1  "XPP_x"
  Integrator4/1 -> [xp_t2], Integrator7/1  "XP_t2"
  Integrator1/1 -> [x_t3]
  [xp_t1] -> Mux1/1
  [x_t2] -> Mux2/2
  Demux/2 -> Integrator4/1  "XPP_t2"
  Demux/1 -> Integrator3/1  "XPP_t1"

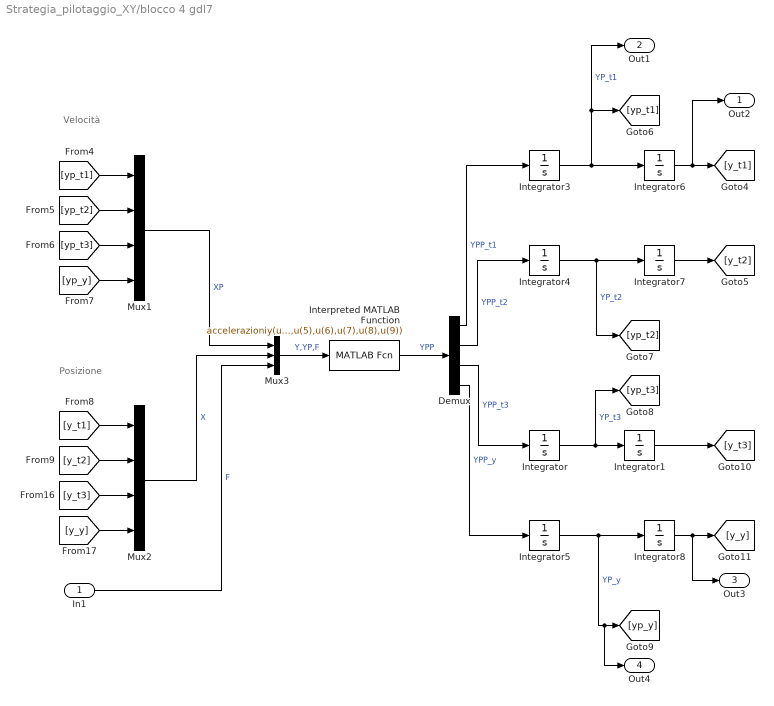
== system Strategia_pilotaggio_XY/blocco 4 gdl7 ==
  note: Posizione
  note: Velocità
  In1 : Inport
  Demux : Demux
  Integrator{,3..5} (4 alike) : Integrator
  Integrator1 : Integrator  InitialCondition=ci_y(3)
  Integrator6 : Integrator  InitialCondition=ci_y(1)
  Integrator7 : Integrator  InitialCondition=ci_y(2)
  Integrator8 : Integrator  InitialCondition=ci_y(4)
  Interpreted MATLAB Function : MATLABFcn  MATLABFcn=accelerazioniy(u(1),u(2),u(3),u(4),u(5),u(6),u(7),u(8),u(9))  OutputDimensions=4
  Mux1 : Mux
  Mux2 : Mux
  Mux3 : Mux  Inputs=3
  Out2 : Outport
  Out1 : Outport  Port=2
  Out3 : Outport  Port=3
  Out4 : Outport  Port=4
  wires:
  Integrator/1 -> Integrator1/1, [yp_t3]  "YP_t3"
  Mux1/1 -> Mux3/1  "XP"
  [y_t3] -> Mux2/3
  Mux3/1 -> Interpreted MATLAB Function/1  "Y,YP,F"
  [y_t2] -> Mux2/2
  Integrator7/1 -> [y_t2]
  Demux/3 -> Integrator/1  "YPP_t3"
  [yp_y] -> Mux1/4
  [y_y] -> Mux2/4
  Demux/1 -> Integrator3/1  "YPP_t1"
  [yp_t2] -> Mux1/2
  Mux2/1 -> Mux3/2  "X"
  Interpreted MATLAB Function/1 -> Demux/1  "YPP"
  Integrator8/1 -> Out3/1, [y_y]
  Integrator4/1 -> [yp_t2], Integrator7/1  "YP_t2"
  Integrator3/1 -> Out1/1, [yp_t1], Integrator6/1  "YP_t1"
  In1/1 -> Mux3/3  "F"
  Demux/2 -> Integrator4/1  "YPP_t2"
  Integrator5/1 -> Out4/1, [yp_y], Integrator8/1  "YP_y"
  Integrator6/1 -> Out2/1, [y_t1]
  [yp_t3] -> Mux1/3
  Demux/4 -> Integrator5/1  "YPP_y"
  Integrator1/1 -> [y_t3]
  [yp_t1] -> Mux1/1
  [y_t1] -> Mux2/1

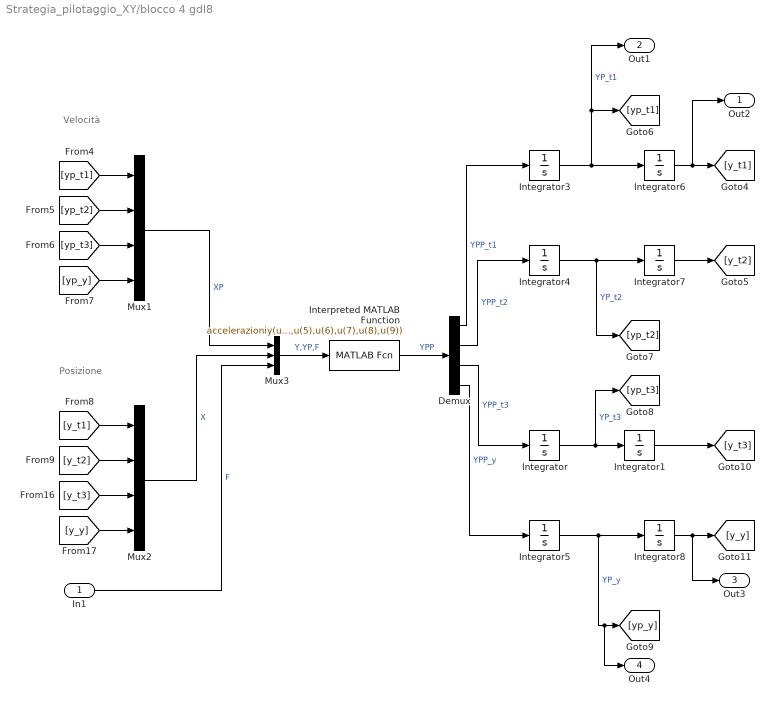
== system Strategia_pilotaggio_XY/blocco 4 gdl8 ==
  note: Posizione
  note: Velocità
  In1 : Inport
  Demux : Demux
  Integrator{,3..5} (4 alike) : Integrator
  Integrator1 : Integrator  InitialCondition=ci_y(3)
  Integrator6 : Integrator  InitialCondition=ci_y(1)
  Integrator7 : Integrator  InitialCondition=ci_y(2)
  Integrator8 : Integrator  InitialCondition=ci_y(4)
  Interpreted MATLAB Function : MATLABFcn  MATLABFcn=accelerazioniy(u(1),u(2),u(3),u(4),u(5),u(6),u(7),u(8),u(9))  OutputDimensions=4
  Mux1 : Mux
  Mux2 : Mux
  Mux3 : Mux  Inputs=3
  Out2 : Outport
  Out1 : Outport  Port=2
  Out3 : Outport  Port=3
  Out4 : Outport  Port=4
  wires:
  Integrator/1 -> Integrator1/1, [yp_t3]  "YP_t3"
  Mux1/1 -> Mux3/1  "XP"
  [y_t3] -> Mux2/3
  Mux3/1 -> Interpreted MATLAB Function/1  "Y,YP,F"
  [y_t2] -> Mux2/2
  Integrator7/1 -> [y_t2]
  Demux/3 -> Integrator/1  "YPP_t3"
  [yp_y] -> Mux1/4
  [y_y] -> Mux2/4
  Demux/1 -> Integrator3/1  "YPP_t1"
  [yp_t2] -> Mux1/2
  Mux2/1 -> Mux3/2  "X"
  Interpreted MATLAB Function/1 -> Demux/1  "YPP"
  Integrator8/1 -> Out3/1, [y_y]
  Integrator4/1 -> [yp_t2], Integrator7/1  "YP_t2"
  Integrator3/1 -> Out1/1, [yp_t1], Integrator6/1  "YP_t1"
  In1/1 -> Mux3/3  "F"
  Demux/2 -> Integrator4/1  "YPP_t2"
  Integrator5/1 -> Out4/1, [yp_y], Integrator8/1  "YP_y"
  Integrator6/1 -> Out2/1, [y_t1]
  [yp_t3] -> Mux1/3
  Demux/4 -> Integrator5/1  "YPP_y"
  Integrator1/1 -> [y_t3]
  [yp_t1] -> Mux1/1
  [y_t1] -> Mux2/1
